simulink model "Prescan_Carsim_1110_cs"  (R2019b)
settings: Solver=ode5  StartTime=0.0  StopTime=inf  FixedStep=1/20  RelTol=1e-3
PreLoadFcn:
  | mbxruntime.callbacks.PreLoadFcn(bdroot);
PostLoadFcn:
  | mbxruntime.callbacks.PostLoadFcn(bdroot);
InitFcn:
  | mbxruntime.callbacks.InitFcn(bdroot);
  | Initialization_Func;
  | %T01_Init_2106;
StartFcn:
  | mbxruntime.callbacks.StartFcn(bdroot);
  | current_sys=gcs;
  | speedblock=Simulink.findBlocks(current_sys,'Name','speed_kmh_Gain');
  | h1=add_exec_event_listener(speedblock,'PostOutputs',@SpeedVisulization);
  | outblock=Simulink.findBlocks(current_sys,'Name','trajectorycurveoutput_Gain');
  | CurveTrajectoryListenerHandle=add_exec_event_listener(outblock,'PostOutputs',@TrajectoryCurve_CallBack);
  | lanedatablock=Simulink.findBlocks(current_sys,'Name','LaneData_Gain');
  | CurveLaneListenerHandle=add_exec_event_listener(lanedatablock,'PostOutputs',@CurveLane_CallBack);
StopFcn:
  | mbxruntime.callbacks.StopFcn(bdroot);
model workspace: external: MAT-File .\Prescan_Carsim_1110_cs_hws.mat (data not in the file)
undefined symbols (not defined in the file): AAx, AAy, AAz, AVx, AVy, AVz, Ax, Ay, Az, canChannel, DiscIntNeverNeededParam, g, InitialDPMPDF_Comfort, InitialDPMPDF_Efficiency, InitialDPMPDF_Safety, InitialPDF_DEM, InitialPlanningParameter, Kf, Kr, Lr, M, mbxruntime, nG, NormalisedTrajectoryIndicator_Pool, Parameter_Indicator_LookUpTable, Prescan_Carsim_1110_cs_119509d653dbd015, Prescan_Carsim_1110_cs_2a185a1795bc1743, Prescan_Carsim_1110_cs_518c510c1da40fb3, Prescan_Carsim_1110_cs_52de4d8fa74bbcb1, Prescan_Carsim_1110_cs_b8364abf183e6ec6, Prescan_Carsim_1110_cs_fca2a77e3ded9ac6, Rational_Coefficient_Learning, SteeringWheel, TrajectoryIndicatorRange, V, VehicleBaseLength, Vx, Vy, Vz
libraries: canmsglib x11, dsparch4 x5, canlib x3, PreScanSimulinkLibrary x3, Solver_SF x1, autolibshared x1
(part 3 of 6)

== system Prescan_Carsim_1110_cs/BMW_X5_SUV_1/LaneMarkerSensor_1_Data/If Action Subsystem2 ==
  In1 : Inport
  In2 : Inport  Port=2
  Action Port : ActionPort  ActionPortLabel=if(u1 >= u2)
  Bus Selector : BusSelector  OutputSignals=DATA
  Selector : Selector  IndexOptions=Index vector (port)  Indices=[4]  OutputSizes=1
  Out1 : Outport
  wires:
  Bus Selector/1 -> Out1/1  "<DATA>"
  Selector/1 -> Bus Selector/1
  In1/1 -> Selector/1
  In2/1 -> Selector/2

== system Prescan_Carsim_1110_cs/BMW_X5_SUV_1/LaneMarkerSensor_1_Data/If Action Subsystem3 ==
  In1 : Inport
  In2 : Inport  Port=2
  Action Port : ActionPort  ActionPortLabel=if(u1 >= u2)
  Bus Selector : BusSelector  OutputSignals=DATA
  Selector : Selector  IndexOptions=Index vector (port)  Indices=[4]  OutputSizes=1
  Out1 : Outport
  wires:
  Bus Selector/1 -> Out1/1  "<DATA>"
  Selector/1 -> Bus Selector/1
  In1/1 -> Selector/1
  In2/1 -> Selector/2

== system Prescan_Carsim_1110_cs/BMW_X5_SUV_1/LaneMarkerSensor_1_Data/If Action Subsystem4 ==
  In1 : Inport
  In2 : Inport  Port=2
  Action Port : ActionPort  ActionPortLabel=if(u1 >= u2)
  Bus Selector : BusSelector  OutputSignals=DATA
  Selector : Selector  IndexOptions=Index vector (port)  Indices=[4]  OutputSizes=1
  Out1 : Outport
  wires:
  Bus Selector/1 -> Out1/1  "<DATA>"
  Selector/1 -> Bus Selector/1
  In1/1 -> Selector/1
  In2/1 -> Selector/2

== system Prescan_Carsim_1110_cs/BMW_X5_SUV_1/SELF_Demux/compas converter ==
  rotz [rad] : Inport
  cart2compas : Subsystem
  rad2deg : Gain  Gain=180/pi
  heading [deg] : Outport
  wires:
  rad2deg/1 -> cart2compas/1(Angle [deg])
  rotz [rad]/1 -> rad2deg/1
  cart2compas/1(heading [deg]) -> heading [deg]/1

== system Prescan_Carsim_1110_cs/BMW_X5_SUV_1/Tracking Control & vehicle dynamics/Lane Keeping Assistance ==
  note: Trajectory Trackin-LQR controller, Carsim Model
  note: Trajectory Trackin-LQR controller, Simulink VDM
  note: Trajectory Tracking Controller-SMC controller
  DataUsedForTracking (PrescanToTarget)t : Inport
  Bus Selector : BusSelector  OutputSignals=Preview Error,HeadError_rad,Curvature,PreviewDistance,Speed_Kmh
  Digital Filter Design6 : dsparch4/Digital Filter Design  Commented=on  mwdsp_browser_bugfix_var=off
  From : From  Commented=on  GotoTag=SMC_c1  TagVisibility=global
  From1 : From  Commented=on  GotoTag=SMC_c2  TagVisibility=global
  From3 : From  Commented=on  GotoTag=delta  TagVisibility=global
  From4 : From  Commented=on  GotoTag=kapa  TagVisibility=global
  Gain : Gain  Gain=180/pi
  Gain1 : Gain  Gain=1/3.6
  Manual Switch : ManualSwitch  CurrentSetting=0
  Manual Switch1 : ManualSwitch  CurrentSetting=0
  Path Tracking - LQR controller : Subsystem  Commented=on
  Path Tracking - LQR controller1 : Subsystem
  Path Tracking - SMC controller : MATLAB Function  Commented=on  TreatAsAtomicUnit=on
  SMC characters : Subsystem  Commented=on
  derivative_filter : Subsystem
  "derivative_filter " : Subsystem
  steering angle_Front(deg) : Outport
  wires:
  Path Tracking - LQR controller/1(SteeringAngle_Front(rad)) -> Manual Switch1/1
  Gain1/1 -> Path Tracking - LQR controller1/7(Speed_m/s), Path Tracking - LQR controller/7(Speed_m/s), Path Tracking - SMC controller/11(v)
  Gain/1 -> steering angle_Front(deg)/1
  "derivative_filter "/1(Out1) -> Path Tracking - LQR controller1/2(PreviewError_dot), Path Tracking - LQR controller/2(PreviewError_dot), Path Tracking - SMC controller/6(PreviewError_dot)
  Digital Filter Design6/1 -> Manual Switch/1  "steering angle"
  From/1 -> Path Tracking - SMC controller/1(c1)
  derivative_filter/1(Out1) -> Path Tracking - LQR controller1/4(HeadingError_dot), Path Tracking - LQR controller/4(HeadingError_dot), Path Tracking - SMC controller/8(HeadingError_dot)
  Path Tracking - SMC controller/1(SteerAngle) -> Digital Filter Design6/1
  From3/1 -> Path Tracking - SMC controller/3(delta)
  From1/1 -> Path Tracking - SMC controller/2(c2)
  From4/1 -> Path Tracking - SMC controller/4(kapa)
  Bus Selector/5 -> Gain1/1  "<Speed_Kmh>"
  Bus Selector/1 -> Path Tracking - SMC controller/5(PreviewError), Path Tracking - LQR controller1/1(PreviewError), Path Tracking - LQR controller/1(PreviewError), "derivative_filter "/1(In1)  "<Preview Error>"
  Bus Selector/4 -> Path Tracking - SMC controller/10(PreviewDistance), Path Tracking - LQR controller1/6(Preview_Distance), Path Tracking - LQR controller/6(Preview_Distance)  "<PreviewDistance>"
  Bus Selector/2 -> Path Tracking - LQR controller1/3(HeadingError), Path Tracking - LQR controller/3(HeadingError), Path Tracking - SMC controller/7(HeadingError), derivative_filter/1(In1)  "<HeadError_rad>"
  Manual Switch/1 -> Gain/1
  Bus Selector/3 -> Path Tracking - LQR controller1/5(Curvature), Path Tracking - LQR controller/5(Curvature), Path Tracking - SMC controller/9(Curvature)  "<Curvature>"
  DataUsedForTracking (PrescanToTarget)t/1 -> Bus Selector/1
  Path Tracking - LQR controller1/1(SteeringAngle_Front(rad)) -> Manual Switch1/2
  Manual Switch1/1 -> Manual Switch/2

== system Prescan_Carsim_1110_cs/BMW_X5_SUV_1/Tracking Control & vehicle dynamics/simple_filter10 ==
  In1 : Inport
  Add : Sum
  Gain10 : Gain  Gain=0.5
  Memory : Memory
  Out1 : Outport  VectorParamsAs1DForOutWhenUnconnected=off
  wires:
  Gain10/1 -> Out1/1
  Memory/1 -> Add/2
  In1/1 -> Add/1, Memory/1
  Add/1 -> Gain10/1

== system Prescan_Carsim_1110_cs/BMW_X5_SUV_1/Tracking Control & vehicle dynamics/simple_filter11 ==
  In1 : Inport
  Add : Sum
  Gain10 : Gain  Gain=0.5
  Memory : Memory
  Out1 : Outport  VectorParamsAs1DForOutWhenUnconnected=off
  wires:
  Gain10/1 -> Out1/1
  Memory/1 -> Add/2
  In1/1 -> Add/1, Memory/1
  Add/1 -> Gain10/1

== system Prescan_Carsim_1110_cs/BMW_X5_SUV_1/Tracking Control & vehicle dynamics/simple_filter6 ==
  In1 : Inport
  Add : Sum
  Gain10 : Gain  Gain=0.5
  Memory : Memory
  Out1 : Outport  VectorParamsAs1DForOutWhenUnconnected=off
  wires:
  Add/1 -> Gain10/1
  In1/1 -> Memory/1, Add/1
  Memory/1 -> Add/2
  Gain10/1 -> Out1/1

== system Prescan_Carsim_1110_cs/BMW_X5_SUV_1/Tracking Control & vehicle dynamics/simple_filter7 ==
  In1 : Inport
  Add : Sum
  Gain10 : Gain  Gain=0.5
  Memory : Memory
  Out1 : Outport  VectorParamsAs1DForOutWhenUnconnected=off
  wires:
  Gain10/1 -> Out1/1
  Memory/1 -> Add/2
  In1/1 -> Add/1, Memory/1
  Add/1 -> Gain10/1

== system Prescan_Carsim_1110_cs/BMW_X5_SUV_1/Tracking Control & vehicle dynamics/simple_filter8 ==
  In1 : Inport
  Add : Sum
  Gain10 : Gain  Gain=0.5
  Memory : Memory
  Out1 : Outport  VectorParamsAs1DForOutWhenUnconnected=off
  wires:
  Add/1 -> Gain10/1
  In1/1 -> Memory/1, Add/1
  Memory/1 -> Add/2
  Gain10/1 -> Out1/1

== system Prescan_Carsim_1110_cs/BMW_X5_SUV_1/Tracking Control & vehicle dynamics/simple_filter9 ==
  In1 : Inport
  Add : Sum
  Gain10 : Gain  Gain=0.5
  Memory : Memory
  Out1 : Outport  VectorParamsAs1DForOutWhenUnconnected=off
  wires:
  Gain10/1 -> Out1/1
  Memory/1 -> Add/2
  In1/1 -> Add/1, Memory/1
  Add/1 -> Gain10/1

== system Prescan_Carsim_1110_cs/BMW_X5_SUV_1/Trajectory Indicator Calculation/VehicleInfo_Curve ==
  In1 : Inport
  Trigger : TriggerPort  TriggerType=falling  VariantControl=Variant
  trajectorycurveoutput_Gain : Gain
  VehicleInfo_Curve : Outport
  wires:
  In1/1 -> trajectorycurveoutput_Gain/1
  trajectorycurveoutput_Gain/1 -> VehicleInfo_Curve/1

== system Prescan_Carsim_1110_cs/BMW_X5_SUV_1/Trajectory Indicator Calculation/VehicleState_Buffer ==
  In1 : Inport
  Enable : EnablePort  StatesWhenEnabling=reset  PropagateVarSize=During execution
  VehicleInfo_StoreDuringCurve : MATLAB Function  TreatAsAtomicUnit=on
  VehicleInfo_Curve : Outport
  wires:
  In1/1 -> VehicleInfo_StoreDuringCurve/1(VehicleState_Var)
  VehicleInfo_StoreDuringCurve/1(VehicleState_Curve) -> VehicleInfo_Curve/1

== system Prescan_Carsim_1110_cs/BMW_X5_SUV_1/VehicleToPrescan/simple_filter10 ==
  In1 : Inport
  Add : Sum
  Gain10 : Gain  Gain=0.5
  Memory : Memory
  Out1 : Outport  VectorParamsAs1DForOutWhenUnconnected=off
  wires:
  Gain10/1 -> Out1/1
  Memory/1 -> Add/2
  In1/1 -> Add/1, Memory/1
  Add/1 -> Gain10/1

== system Prescan_Carsim_1110_cs/BMW_X5_SUV_1/VehicleToPrescan/simple_filter11 ==
  In1 : Inport
  Add : Sum
  Gain10 : Gain  Gain=0.5
  Memory : Memory
  Out1 : Outport  VectorParamsAs1DForOutWhenUnconnected=off
  wires:
  Gain10/1 -> Out1/1
  Memory/1 -> Add/2
  In1/1 -> Add/1, Memory/1
  Add/1 -> Gain10/1

== system Prescan_Carsim_1110_cs/BMW_X5_SUV_1/VehicleToPrescan/simple_filter6 ==
  In1 : Inport
  Add : Sum
  Gain10 : Gain  Gain=0.5
  Memory : Memory
  Out1 : Outport  VectorParamsAs1DForOutWhenUnconnected=off
  wires:
  Add/1 -> Gain10/1
  In1/1 -> Memory/1, Add/1
  Memory/1 -> Add/2
  Gain10/1 -> Out1/1

== system Prescan_Carsim_1110_cs/BMW_X5_SUV_1/VehicleToPrescan/simple_filter7 ==
  In1 : Inport
  Add : Sum
  Gain10 : Gain  Gain=0.5
  Memory : Memory
  Out1 : Outport  VectorParamsAs1DForOutWhenUnconnected=off
  wires:
  Gain10/1 -> Out1/1
  Memory/1 -> Add/2
  In1/1 -> Add/1, Memory/1
  Add/1 -> Gain10/1

== system Prescan_Carsim_1110_cs/BMW_X5_SUV_1/VehicleToPrescan/simple_filter8 ==
  In1 : Inport
  Add : Sum
  Gain10 : Gain  Gain=0.5
  Memory : Memory
  Out1 : Outport  VectorParamsAs1DForOutWhenUnconnected=off
  wires:
  Add/1 -> Gain10/1
  In1/1 -> Memory/1, Add/1
  Memory/1 -> Add/2
  Gain10/1 -> Out1/1

== system Prescan_Carsim_1110_cs/BMW_X5_SUV_1/VehicleToPrescan/simple_filter9 ==
  In1 : Inport
  Add : Sum
  Gain10 : Gain  Gain=0.5
  Memory : Memory
  Out1 : Outport  VectorParamsAs1DForOutWhenUnconnected=off
  wires:
  Gain10/1 -> Out1/1
  Memory/1 -> Add/2
  In1/1 -> Add/1, Memory/1
  Add/1 -> Gain10/1

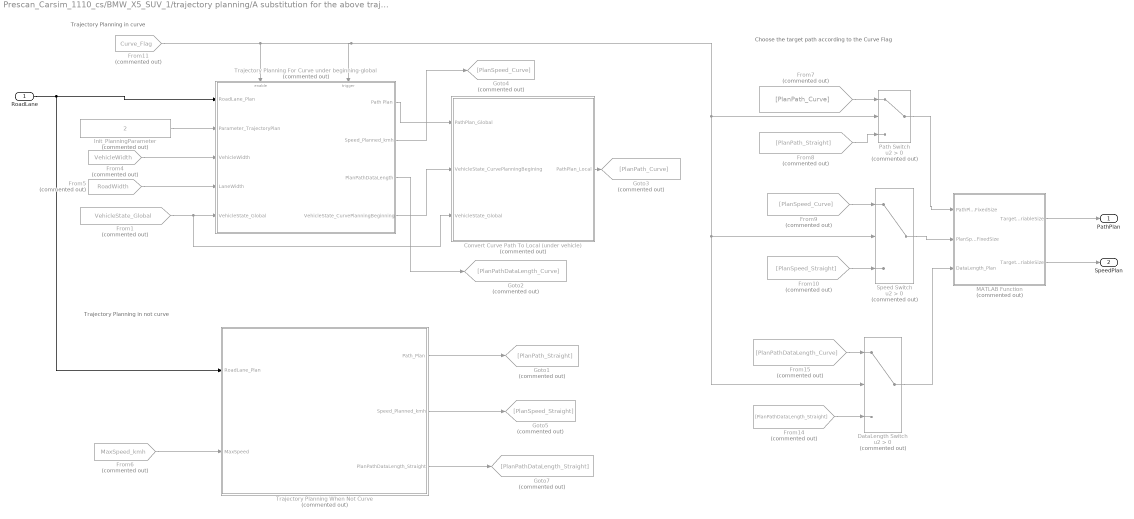
== system Prescan_Carsim_1110_cs/BMW_X5_SUV_1/trajectory planning/A substitution for the above trajectory planning subsystem ==
  note: Choose the target path according to the Curve Flag
  note: Trajectory Planning in not curve
  note: Trajectory Planning in curve
  RoadLane : Inport
  Convert Curve Path To Local (under vehicle) : MATLAB Function  Commented=on  TreatAsAtomicUnit=on
  DataLength Switch : Switch  Commented=on  Criteria=u2 > Threshold
  From1 : From  Commented=on  GotoTag=VehicleState_Global  TagVisibility=global
  From10 : From  Commented=on  GotoTag=PlanSpeed_Straight
  From11 : From  Commented=on  GotoTag=Curve_Flag  TagVisibility=global
  From14 : From  Commented=on  GotoTag=PlanPathDataLength_Straight
  From15 : From  Commented=on  GotoTag=PlanPathDataLength_Curve
  From4 : From  Commented=on  GotoTag=VehicleWidth  TagVisibility=global
  From5 : From  Commented=on  GotoTag=RoadWidth  TagVisibility=global
  From6 : From  Commented=on  GotoTag=MaxSpeed_kmh  TagVisibility=global
  From7 : From  Commented=on  GotoTag=PlanPath_Curve
  From8 : From  Commented=on  GotoTag=PlanPath_Straight
  From9 : From  Commented=on  GotoTag=PlanSpeed_Curve
  Goto1 : Goto  Commented=on  GotoTag=PlanPath_Straight
      settings: AttributesFormatString=output:fixed size,1000*2
  Goto2 : Goto  Commented=on  GotoTag=PlanPathDataLength_Curve
  Goto3 : Goto  Commented=on  GotoTag=PlanPath_Curve
      settings: AttributesFormatString=|
      | Path local under the vehicle
      | output:fixed size 1000*2
  Goto4 : Goto  Commented=on  GotoTag=PlanSpeed_Curve
      settings: AttributesFormatString=The size is fixed 1000*1
  Goto5 : Goto  Commented=on  GotoTag=PlanSpeed_Straight
      settings: AttributesFormatString=The size vas fixed 1000*1
  Goto7 : Goto  Commented=on  GotoTag=PlanPathDataLength_Straight
      settings: AttributesFormatString=|
      | Used to extract the valid
      | PlanPath data
  Init_PlanningParameter : Constant  Commented=on  Value=2
  MATLAB Function : MATLAB Function  Commented=on  TreatAsAtomicUnit=on  SystemSampleTime=1/20
      settings: AttributesFormatString=|
      | Convert Variable Size into Fixed Size
      | Specified Sample Time:1/20
  Path Switch : Switch  Commented=on  Criteria=u2 > Threshold
  Speed Switch : Switch  Commented=on  Criteria=u2 > Threshold
  Trajectory Planning For Curve under beginning-global : Subsystem  Commented=on
  Trajectory Planning When Not Curve : MATLAB Function  Commented=on  TreatAsAtomicUnit=on
  PathPlan : Outport
  SpeedPlan : Outport  Port=2
  wires:
  From9/1 -> Speed Switch/1
  From11/1 -> Trajectory Planning For Curve under beginning-global/Trigger, Speed Switch/2, DataLength Switch/2, Path Switch/2, Trajectory Planning For Curve under beginning-global/Enable
  Trajectory Planning For Curve under beginning-global/2(Speed_Planned_kmh) -> Goto4/1
  From15/1 -> DataLength Switch/1
  Path Switch/1 -> MATLAB Function/1(PathPlan_FixedSize)
  DataLength Switch/1 -> MATLAB Function/3(DataLength_Plan)
  From10/1 -> Speed Switch/3
  From14/1 -> DataLength Switch/3
  From8/1 -> Path Switch/3
  Speed Switch/1 -> MATLAB Function/2(PlanSpeed_FixedSize)
  Trajectory Planning When Not Curve/3(PlanPathDataLength_Straight) -> Goto7/1
  Trajectory Planning For Curve under beginning-global/3(PlanPathDataLength) -> Goto2/1
  Trajectory Planning For Curve under beginning-global/1(Path Plan) -> Convert Curve Path To Local (under vehicle)/1(PathPlan_Global)
  From1/1 -> Trajectory Planning For Curve under beginning-global/5(VehicleState_Global), Convert Curve Path To Local (under vehicle)/3(VehicleState_Global)
  Trajectory Planning For Curve under beginning-global/4(VehicleState_CurvePlanningBeginning) -> Convert Curve Path To Local (under vehicle)/2(VehicleState_CurvePlanningBegining)
  Init_PlanningParameter/1 -> Trajectory Planning For Curve under beginning-global/2(Parameter_TrajectoryPlan)
  RoadLane/1 -> Trajectory Planning When Not Curve/1(RoadLane_Plan), Trajectory Planning For Curve under beginning-global/1(RoadLane_Plan)
  Trajectory Planning When Not Curve/2(Speed_Planned_kmh) -> Goto5/1
  From7/1 -> Path Switch/1
  From5/1 -> Trajectory Planning For Curve under beginning-global/4(LaneWidth)
  From4/1 -> Trajectory Planning For Curve under beginning-global/3(VehicleWidth)
  Trajectory Planning When Not Curve/1(Path_Plan) -> Goto1/1
  Convert Curve Path To Local (under vehicle)/1(PathPlan_Local) -> Goto3/1
  From6/1 -> Trajectory Planning When Not Curve/2(MaxSpeed)
  MATLAB Function/1(TargetPath_VariableSize) -> PathPlan/1
  MATLAB Function/2(TargetSpeed_VariableSize) -> SpeedPlan/1

== system Prescan_Carsim_1110_cs/BMW_X5_SUV_1/trajectory planning/Generate Road Lane from Polyfit TLC calculation  ==
  PolyRoadLane : Inport
  RoadLaneEnd_Rotation : Inport  Port=2
  Mux : Mux  Inputs=2
  Pre_Dis : Constant  Value=150
      settings: AttributesFormatString=The Preview Distance used to calculate the TLC
  Scope : Scope
  "TLC calculation and Lane Generation Road Lane " : MATLAB Function  TreatAsAtomicUnit=on
      settings: AttributesFormatString=|
      | The TLC could not be calculated because
      | of the optimal function is not available
      | for simulink code generation
  Terminator : Terminator
  tag scope: TLC_Left=global, TLC_Right=global
  wires:
  PolyRoadLane/1 -> "TLC calculation and Lane Generation Road Lane "/1(PolyRoadLane)
  "TLC calculation and Lane Generation Road Lane "/2(TLC_Left) -> Mux/1, [TLC_Left]
  [Interval_RoadSegment] -> "TLC calculation and Lane Generation Road Lane "/3(IntervalRoadSegment)
  RoadLaneEnd_Rotation/1 -> "TLC calculation and Lane Generation Road Lane "/2(RoadLaneEnd_Rotation)
  [RoadWidth] -> "TLC calculation and Lane Generation Road Lane "/4(Width_Road)
  [VehicleWidth] -> "TLC calculation and Lane Generation Road Lane "/5(Width_Vehicle)
  Pre_Dis/1 -> "TLC calculation and Lane Generation Road Lane "/7(Range)
  [VehicleBaseLength] -> "TLC calculation and Lane Generation Road Lane "/6(Length_Vehicle)
  [YawRate] -> "TLC calculation and Lane Generation Road Lane "/8(YawRate)
  [Speed_Rel] -> "TLC calculation and Lane Generation Road Lane "/9(Speed)
  "TLC calculation and Lane Generation Road Lane "/3(TLC_Right) -> Mux/2, [TLC_Right]
  "TLC calculation and Lane Generation Road Lane "/1(RoadLane_Plan) -> Terminator/1
  Mux/1 -> Scope/1

== system Prescan_Carsim_1110_cs/BMW_X5_SUV_1/trajectory planning/Out of Specific Curve Planning ==
  RoadLane_Plan : Inport
  MaxSpeed_Kmh : Inport  Port=2
  Action Port : ActionPort  ActionPortLabel=else
  Trajectory Planning When Not Curve : MATLAB Function  TreatAsAtomicUnit=on
  Path Plan : Outport
  Speed_Planned_kmh : Outport  Port=2
  PlanPathDataLength : Outport  Port=3
  wires:
  RoadLane_Plan/1 -> Trajectory Planning When Not Curve/1(RoadLane_Plan)
  Trajectory Planning When Not Curve/1(Path_Plan) -> Path Plan/1
  Trajectory Planning When Not Curve/2(Speed_Planned_kmh) -> Speed_Planned_kmh/1
  Trajectory Planning When Not Curve/3(PlanPathDataLength_Straight) -> PlanPathDataLength/1
  MaxSpeed_Kmh/1 -> Trajectory Planning When Not Curve/2(MaxSpeed)

== system Prescan_Carsim_1110_cs/BMW_X5_SUV_1/trajectory planning/Specific Curve Trajectory Planning ==
  CurveFlag : Inport
  RoadLane_Plan : Inport  Port=2
  PlanningParameter : Inport  Port=3
  VehicleWidth : Inport  Port=4
  LaneWidth : Inport  Port=5
  VehicleState_Global : Inport  Port=6
  Action Port : ActionPort  InitializeStates=reset  PropagateVarSize=During execution  ActionPortLabel=if(u1 > 0)
  Convert Curve Path To Local (under vehicle) : MATLAB Function  TreatAsAtomicUnit=on
  Trajectory Planning For Curve under beginning-global : Subsystem
  Path Plan : Outport
  Speed_Planned_kmh : Outport  Port=2
  PlanPathDataLength : Outport  Port=3
  wires:
  CurveFlag/1 -> Trajectory Planning For Curve under beginning-global/Trigger
  Trajectory Planning For Curve under beginning-global/1(Path Plan) -> Convert Curve Path To Local (under vehicle)/1(PathPlan_Global)
  Convert Curve Path To Local (under vehicle)/1(PathPlan_Local) -> Path Plan/1
  Trajectory Planning For Curve under beginning-global/2(Speed_Planned_kmh) -> Speed_Planned_kmh/1
  Trajectory Planning For Curve under beginning-global/3(PlanPathDataLength) -> PlanPathDataLength/1
  RoadLane_Plan/1 -> Trajectory Planning For Curve under beginning-global/1(RoadLane_Plan)
  VehicleState_Global/1 -> Trajectory Planning For Curve under beginning-global/5(VehicleState_Global), Convert Curve Path To Local (under vehicle)/2(VehicleState_Global)
  VehicleWidth/1 -> Trajectory Planning For Curve under beginning-global/3(VehicleWidth)
  LaneWidth/1 -> Trajectory Planning For Curve under beginning-global/4(LaneWidth)
  PlanningParameter/1 -> Trajectory Planning For Curve under beginning-global/2(Parameter_TrajectoryPlan)

== system Prescan_Carsim_1110_cs/BMW_X5_SUV_1/trajectory planning/Subsystem ==
  Choose curve length for different curve No : MultiPortSwitch  Inputs=4  DataPortForDefault=Additional data port  DiagnosticForDefault=None
  Constant : Constant
  Constant1 : Constant  Value=0
  "Curve 1 " : Constant  Value=308
  Curve 2 : Constant  Value=308
  Curve 3 : Constant  Value=308
  Curve 4 : Constant  Value=308
  Determination of Curve Road No : Subsystem
  Not Curve : Constant  Value=160
  Sum : Sum  Inputs=2
  Switch : Switch  Criteria=u2 > Threshold  Threshold=0.5
  The planned path length after curve : Constant  Value=8
      settings: AttributesFormatString=Should consider the Preview Distance
  Expected PathPlanning Length : Outport
  Curve Flag : Outport  Port=2
      settings: AttributesFormatString=|
      | 1: Curve
      | 0: Not Curve
  wires:
  Determination of Curve Road No/1(Curve No) -> Switch/2, Choose curve length for different curve No/1
  Not Curve/1 -> Choose curve length for different curve No/6
  Curve 4/1 -> Choose curve length for different curve No/5
  Curve 3/1 -> Choose curve length for different curve No/4
  Sum/1 -> Expected PathPlanning Length/1
  Curve 2/1 -> Choose curve length for different curve No/3
  "Curve 1 "/1 -> Choose curve length for different curve No/2
  The planned path length after curve/1 -> Sum/2
  Choose curve length for different curve No/1 -> Sum/1
  Switch/1 -> Curve Flag/1
  Constant/1 -> Switch/1
  Constant1/1 -> Switch/3

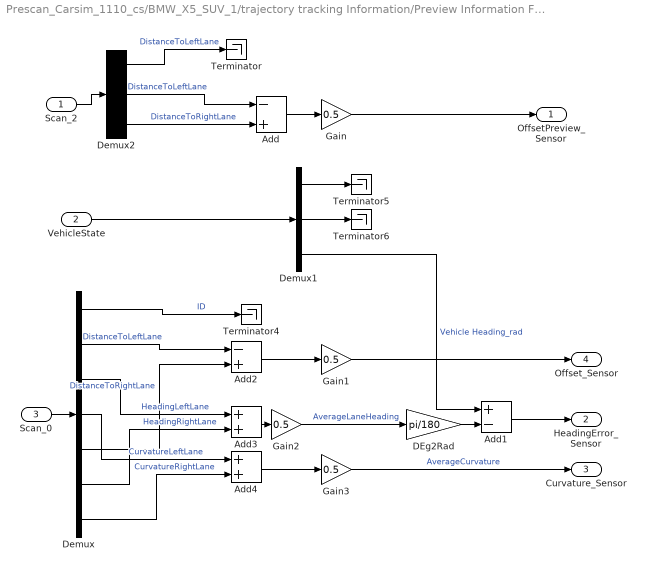
== system Prescan_Carsim_1110_cs/BMW_X5_SUV_1/trajectory tracking Information/Preview Information From LaneMarkerSensor ==
  Scan_2 : Inport
  VehicleState : Inport  Port=2
  Scan_0 : Inport  Port=3
  Add : Sum  Inputs=-+
  Add1 : Sum  Inputs=+-
  Add2 : Sum  Inputs=-+
  Add3 : Sum
  Add4 : Sum
  DEg2Rad : Gain  Gain=pi/180
  Demux : Demux  Outputs=7  BusSelectionMode=on
  Demux1 : Demux  Outputs=3
  Demux2 : Demux  Outputs=3  BusSelectionMode=on
  Gain{,1..3} (4 alike) : Gain  Gain=0.5
  Terminator{,4..6} (4 alike) : Terminator
  OffsetPreview_Sensor : Outport
  HeadingError_Sensor : Outport  Port=2
  Curvature_Sensor : Outport  Port=3
  Offset_Sensor : Outport  Port=4
  wires:
  Add1/1 -> HeadingError_Sensor/1
  Demux1/1 -> Terminator5/1
  VehicleState/1 -> Demux1/1
  Scan_0/1 -> Demux/1
  Demux1/2 -> Terminator6/1
  Scan_2/1 -> Demux2/1
  Demux2/3 -> Add/2  "DistanceToRightLane"
  Demux2/2 -> Add/1  "DistanceToLeftLane"
  Gain/1 -> OffsetPreview_Sensor/1
  Demux1/3 -> Add1/1  "Vehicle Heading_rad"
  Demux/2 -> Add2/1  "DistanceToLeftLane"
  Gain1/1 -> Offset_Sensor/1
  Add2/1 -> Gain1/1
  Demux/1 -> Terminator4/1  "ID"
  Add3/1 -> Gain2/1
  Gain2/1 -> DEg2Rad/1  "AverageLaneHeading"
  Demux/6 -> Add3/2  "HeadingRightLane"
  Demux/7 -> Add4/2  "CurvatureRightLane"
  Demux/5 -> Add2/2  "DistanceToRightLane"
  Demux/4 -> Add4/1  "CurvatureLeftLane"
  Add4/1 -> Gain3/1
  Demux/3 -> Add3/1  "HeadingLeftLane"
  Gain3/1 -> Curvature_Sensor/1  "AverageCurvature"
  Add/1 -> Gain/1
  Demux2/1 -> Terminator/1  "DistanceToLeftLane"
  DEg2Rad/1 -> Add1/2

== system Prescan_Carsim_1110_cs/SteeringWheel_pivot_BMW_X5_SUV_1/Actuator/visu_Rotate ==
  In1 : Inport
  sfun_RPYActuator : S-Function  FunctionName=sfun_RPYActuator  Parameters=SParameter1, SParameter2, SampleTime  SFunctionDeploymentMode=off  EnableBusSupport=off  mask(Legacy Function){SFunctionSpec=void prescan_outputFcn(void ** work1,  PRESCAN_XYZ_DATA u1[1]), SParameter1=UniqueID, SParameter2=uint8([Object3DID 0]), SampleTime=TimeStep, ShowSpec=on}
      mask prompts: SParameter1 "P1:"; SParameter2 "P2:"; SampleTime "Sample time (-1 for inherited):"; ShowSpec "Display function specification"
      mask help:
      | This block allows you to call the legacy functions specified by the following Legacy Code Tool definition:
      | def.SFunctionName = 'sfun_PositionActuator';
      | def.OutputFcnSpec = 'void prescan_outputFcn(void ** work1,  PRESCAN_XYZ_DATA u1[1])';
      | def.StartFcnSpec = 'void prescan_startFcn(void ** work1, uint8 p1[], double p2)';
      | def.TerminateFcnSpec = 'void prescan_terminateFcn(void ** work1)';
      | def.HeaderFiles = {'prescan_positionactuator_data.h', 'prescan_header_data.h', 'prescan_SFunLibrary.h', 'prescan_CreateLogHandler.h', 'prescan_CreateErrorHandler.h'};
      | def.SourceFiles = {'prescan_MexLogHandler.cpp', 'prescan_SimStructErrorHandler.cpp', 'prescan_ConcurrentLogHandler.cpp', 'prescan_ConcurrentErrorHandler.cpp'};
      | def.HostLibFiles = {'sensorinterfaced.lib'};
      | def.TargetLibFiles = {'sensorinterfaced.so'};
      | def.IncPaths = {'.', 'C:\prescandev\vislibrary\vis\..\pimp\include\sensors\InterfaceRTW'};
      | def.SrcPaths = {'.'};
      | def.LibPaths = {'C:\\prescandev\\vislibrary_build\lib'};
      | def.SampleTime = 'parameterized';
      mask Help: <p>This block was generated automatically by the Legacy Code Tool. For detailed help on this tool, call<a href="matlab:legacy_code('help')"> legacy_code('help')</a>.</p>
      mask Callback ShowSpec:
      | if strcmp(get_param(gcbh, 'ShowSpec'), 'on')
      |   set_param(gcbh, 'MaskDisplay', sprintf('fprintf(''%s'');', get_param(gcbh, 'SFunctionSpec')));
      | else
      |   set_param(gcbh, 'MaskDisplay', sprintf('fprintf(''%s'');', get_param(gcbh, 'FunctionName')));
      | end
      mask Display: fprintf('void prescan_outputFcn(void ** work1,  PRESCAN_XYZ_DATA u1[1])');
  wires:
  In1/1 -> sfun_RPYActuator/1

== system Prescan_Carsim_1110_cs/SteeringWheel_pivot_BMW_X5_SUV_1/Actuator/visu_Translate ==
  In1 : Inport
  sfun_PositionActuator : S-Function  FunctionName=sfun_PositionActuator  Parameters=SParameter1, SParameter2, SampleTime  SFunctionDeploymentMode=off  EnableBusSupport=off  mask(Legacy Function){SFunctionSpec=void prescan_outputFcn(void ** work1,  PRESCAN_XYZ_DATA u1[1]), SParameter1=uint8([Object3DID 0]), SParameter2=UniqueID, SampleTime=TimeStep, ShowSpec=on}
      mask prompts: SParameter1 "P1:"; SParameter2 "P2:"; SampleTime "Sample time (-1 for inherited):"; ShowSpec "Display function specification"
      mask help:
      | This block allows you to call the legacy functions specified by the following Legacy Code Tool definition:
      | def.SFunctionName = 'sfun_PositionActuator';
      | def.OutputFcnSpec = 'void prescan_outputFcn(void ** work1,  PRESCAN_XYZ_DATA u1[1])';
      | def.StartFcnSpec = 'void prescan_startFcn(void ** work1, uint8 p1[], double p2)';
      | def.TerminateFcnSpec = 'void prescan_terminateFcn(void ** work1)';
      | def.HeaderFiles = {'prescan_positionactuator_data.h', 'prescan_header_data.h', 'prescan_SFunLibrary.h', 'prescan_CreateLogHandler.h', 'prescan_CreateErrorHandler.h'};
      | def.SourceFiles = {'prescan_MexLogHandler.cpp', 'prescan_SimStructErrorHandler.cpp', 'prescan_ConcurrentLogHandler.cpp', 'prescan_ConcurrentErrorHandler.cpp'};
      | def.HostLibFiles = {'sensorinterfaced.lib'};
      | def.TargetLibFiles = {'sensorinterfaced.so'};
      | def.IncPaths = {'.', 'C:\prescandev\vislibrary\vis\..\pimp\include\sensors\InterfaceRTW'};
      | def.SrcPaths = {'.'};
      | def.LibPaths = {'C:\\prescandev\\vislibrary_build\lib'};
      | def.SampleTime = 'parameterized';
      mask Help: <p>This block was generated automatically by the Legacy Code Tool. For detailed help on this tool, call<a href="matlab:legacy_code('help')"> legacy_code('help')</a>.</p>
      mask Callback ShowSpec:
      | if strcmp(get_param(gcbh, 'ShowSpec'), 'on')
      |   set_param(gcbh, 'MaskDisplay', sprintf('fprintf(''%s'');', get_param(gcbh, 'SFunctionSpec')));
      | else
      |   set_param(gcbh, 'MaskDisplay', sprintf('fprintf(''%s'');', get_param(gcbh, 'FunctionName')));
      | end
      mask Display: fprintf('void prescan_outputFcn(void ** work1,  PRESCAN_XYZ_DATA u1[1])');
  wires:
  In1/1 -> sfun_PositionActuator/1

== system Prescan_Carsim_1110_cs/BMW_X5_SUV_1/DEM updating and Preference Estimation/UpdateDEM/Construct Comparison Group ==
  FeedBack_FromDriver : Inport
  TrajectoryIndicator : Inport  Port=2
  Comparison Group_1 : MATLAB Function  TreatAsAtomicUnit=on
  Constant : Constant  Value=NormalisedTrajectoryIndicator_Pool
  Constant7 : Constant  Value=TrajectoryIndicatorRange
  FeedBack : Outport
  Query_Normalized : Outport  Port=2
  Evaluated_NormlisedTrajectoryIndicator : Outport  Port=3
  LastPreference_Normalised : Outport  Port=4
  wires:
  Comparison Group_1/2(Query_Compare) -> Query_Normalized/1
  FeedBack_FromDriver/1 -> Comparison Group_1/1(Feedback_Driver)
  TrajectoryIndicator/1 -> Comparison Group_1/2(Real_Trajectory_Indicator)
  Constant7/1 -> Comparison Group_1/3(TrajectoryIndicatorRange)
  Constant/1 -> Comparison Group_1/4(NormalisedTrajectoryIndicator_Pool)
  Comparison Group_1/1(FeedBack) -> FeedBack/1
  Comparison Group_1/3(Evaluated_NormalisedTrajectoryIndicator) -> Evaluated_NormlisedTrajectoryIndicator/1
  Comparison Group_1/4(LastPreference_Normalised) -> LastPreference_Normalised/1

== system Prescan_Carsim_1110_cs/BMW_X5_SUV_1/DEM updating and Preference Estimation/UpdateDEM/Online DEM updating ==
  FeedBack : Inport
  Query_Compare : Inport  Port=2
  PriorPDF_DEM : Inport  Port=3
  PriorDPMPDF_Safety : Inport  Port=4
  PriorDPMPDF_Comfort : Inport  Port=5
  PriorDPMPDF_Efficiency : Inport  Port=6
  Evaluated_Normalised : Inport  Port=7
  LastPreference_NormalisedTrajectoryIndicator : Inport  Port=8
  Constant : Constant  Value=NormalisedTrajectoryIndicator_Pool
  Constant3 : Constant  Value=Rational_Coefficient_Learning
  "Select the Next Trajectory " : MATLAB Function  TreatAsAtomicUnit=on
  UPdate DEM : MATLAB Function  TreatAsAtomicUnit=on
  Next_ExpectedTrajectoryIndicator : Outport
  Next_ExpectedTrajectoryID : Outport  Port=2
  wires:
  FeedBack/1 -> UPdate DEM/1(FeedBack)
  Query_Compare/1 -> UPdate DEM/2(Query)
  PriorPDF_DEM/1 -> UPdate DEM/3(PriorPDF_DEM)
  PriorDPMPDF_Safety/1 -> UPdate DEM/4(PriorDPMPDF_Safety)
  PriorDPMPDF_Comfort/1 -> UPdate DEM/5(PriorDPMPDF_Comfort)
  PriorDPMPDF_Efficiency/1 -> UPdate DEM/6(PriorDPMPDF_Efficiency)
  Constant3/1 -> "Select the Next Trajectory "/8(Rational_Coefficient_Learning), UPdate DEM/7(Rational_Coefficient_Learning)
  UPdate DEM/1(PostPDF_DEM) -> "Select the Next Trajectory "/1(PriorPDF_DEM)
  UPdate DEM/2(PostDPMPDF_Safety) -> "Select the Next Trajectory "/2(PriorDPMPDF_Safety)
  UPdate DEM/3(PostDPMPDF_Comfort) -> "Select the Next Trajectory "/3(PriorDPMPDF_Comfort)
  UPdate DEM/4(PostDPMPDF_Effociency) -> "Select the Next Trajectory "/4(PriorDPMPDF_Efficiency)
  "Select the Next Trajectory "/2(ExpectedNext_QueryID) -> Next_ExpectedTrajectoryID/1
  "Select the Next Trajectory "/1(ExpectedNext_NormalisedTrajectoryIndicator) -> Next_ExpectedTrajectoryIndicator/1
  Constant/1 -> "Select the Next Trajectory "/5(NormalisedTrajectoryIndicator_Pool)
  Evaluated_Normalised/1 -> "Select the Next Trajectory "/6(Evaluated_NormalisedTrajectoryIndicator)
  LastPreference_NormalisedTrajectoryIndicator/1 -> "Select the Next Trajectory "/7(LastPreference_NormalisedTrajectoryIndicator)

== system Prescan_Carsim_1110_cs/BMW_X5_SUV_1/DEM updating and Preference Estimation/UpdateDEM/Trajectory Planning Parameter Management1 ==
  Expected_TrajectoryIndicators : Inport
  ExpectedNext_QueryID : Inport  Port=2
  Constant : Constant  Value=InitialPlanningParameter
  Constant4 : Constant  Value=Parameter_Indicator_LookUpTable
  Determine planning parameter according to the expected TrajectoryIndicators_LookUpTable : MATLAB Function  TreatAsAtomicUnit=on
  From : From  Commented=on  GotoTag=Parameter_Indicator_LookUpTable  TagVisibility=global
  From2 : From  Commented=on  GotoTag=InitialPlanningParameter  TagVisibility=global
  Trajectory parameter : Outport
  wires:
  Expected_TrajectoryIndicators/1 -> Determine planning parameter according to the expected TrajectoryIndicators_LookUpTable/2(unused)
  ExpectedNext_QueryID/1 -> Determine planning parameter according to the expected TrajectoryIndicators_LookUpTable/3(ExpectedNext_QueryID)
  Determine planning parameter according to the expected TrajectoryIndicators_LookUpTable/1(PlanningParameter) -> Trajectory parameter/1
  Constant/1 -> Determine planning parameter according to the expected TrajectoryIndicators_LookUpTable/1(IntialTrajectoryPlanningParameter)
  Constant4/1 -> Determine planning parameter according to the expected TrajectoryIndicators_LookUpTable/4(Parameter_IndicatorLookUpTable)

== system Prescan_Carsim_1110_cs/BMW_X5_SUV_1/DEM updating and Preference Estimation/UpdateDEM/Trajectory Planning Parameter Management2 ==
  Expected_TrajectoryIndicators : Inport
  Next_ExpectedTrajectoryIndicatorID : Inport  Port=2
  Constant4 : Constant  Value=Parameter_Indicator_LookUpTable
  Determine planning parameter according to the expected TrajectoryIndicators_LookUpTable : MATLAB Function  TreatAsAtomicUnit=on
  Trajectory parameter : Outport
  wires:
  Expected_TrajectoryIndicators/1 -> Determine planning parameter according to the expected TrajectoryIndicators_LookUpTable/1(unused)
  Next_ExpectedTrajectoryIndicatorID/1 -> Determine planning parameter according to the expected TrajectoryIndicators_LookUpTable/2(ExpectedNext_QueryID)
  Determine planning parameter according to the expected TrajectoryIndicators_LookUpTable/1(PlanningParameter) -> Trajectory parameter/1
  Constant4/1 -> Determine planning parameter according to the expected TrajectoryIndicators_LookUpTable/3(Parameter_IndicatorLookUpTable)

== system Prescan_Carsim_1110_cs/BMW_X5_SUV_1/DEM updating and Preference Estimation/UpdateDEM/online DPM building preference estimation accordign to feedback ==
  note: DEM-
      | Update the DEM and Estimate the Preference
  feedback : Inport
  Trajectory_Indicators : Inport  Port=2
  " Driver Perception Model preference to trajectory indicator" : Subsystem  Commented=on
  Constant : Constant  Value=NormalisedTrajectoryIndicator_Pool
  Constant1 : Constant  Value=InitialPDF_DEM
      settings: AttributesFormatString=|
      | The Initial probability density Distribution
      | of the S-C-E weight of the DEM
  Constant2 : Constant  Value=InitialDPMPDF_Safety
      settings: AttributesFormatString=|
      | The Initial probability density Distribution
      | of the DPM for S-C-E
  Constant3 : Constant  Value=Rational_Coefficient_Learning
  Constant5 : Constant  Value=InitialDPMPDF_Comfort
      settings: AttributesFormatString=|
      | The Initial probability density Distribution
      | of the DPM for S-C-E
  Constant6 : Constant  Value=InitialDPMPDF_Efficiency
      settings: AttributesFormatString=|
      | The Initial probability density Distribution
      | of the DPM for S-C-E
  Constant7 : Constant  Value=TrajectoryIndicatorRange
  MATLAB Function : MATLAB Function  TreatAsAtomicUnit=on
  Terminator{,1..3} (4 alike) : Terminator
  Expected_TrajectoryIndicators : Outport
  ExpectedNext_QueryID : Outport  Port=2
  wires:
  MATLAB Function/1(ExpectedNext_NormalisedTrajectoryIndicator) -> Expected_TrajectoryIndicators/1
  MATLAB Function/2(ExpectedNext_QueryID) -> ExpectedNext_QueryID/1
  MATLAB Function/6(PostDPMPDF_Effociency) -> Terminator3/1
  MATLAB Function/5(PostDPMPDF_Comfort) -> Terminator2/1
  Constant7/1 -> MATLAB Function/8(TrajectoryIndicatorRange)
  Constant6/1 -> MATLAB Function/7(InitialDPMPDF_Efficiency)
  Constant5/1 -> MATLAB Function/6(InitialDPMPDF_Comfort)
  MATLAB Function/4(PostDPMPDF_Safety) -> Terminator1/1
  MATLAB Function/3(PostPDF_DEM) -> Terminator/1
  Trajectory_Indicators/1 -> MATLAB Function/2(Real_Trajectory_Indicator)
  Constant3/1 -> MATLAB Function/9(Rational_Coefficient_Learning)
  Constant2/1 -> MATLAB Function/5(InitialDPMPDF_Safety)
  Constant1/1 -> MATLAB Function/4(InitialPDF_DEM)
  Constant/1 -> MATLAB Function/3(NormalisedTrajectoryIndicator_Pool)
  feedback/1 -> MATLAB Function/1(FeedBack)

== system Prescan_Carsim_1110_cs/BMW_X5_SUV_1/DriverFeedBack/Generate the FeedBack Obtainment Trigger Signal/Subsystem ==
  In1 : Inport
  Trigger : TriggerPort  TriggerType=falling  VariantControl=Variant  PortDimensions=1
  Beginning Time : Outport
  wires:
  In1/1 -> Beginning Time/1

== system Prescan_Carsim_1110_cs/BMW_X5_SUV_1/SELF_Demux/compas converter/cart2compas ==
  Angle [deg] : Inport
  Constant : Constant  Value=90
  Constant1 : Constant  Value=360
  Gain : Gain  Gain=1/360
  Gain1 : Gain  Gain=360
  Gain2 : Gain  Gain=-1
  Rounding Function : Rounding
  Sum : Sum  Inputs=|-+
  Sum1 : Sum  Inputs=-+|
  Sum2 : Sum  Inputs=++|
  heading [deg] : Outport
  wires:
  Gain/1 -> Rounding Function/1
  Rounding Function/1 -> Gain1/1
  Gain1/1 -> Sum/1
  Angle [deg]/1 -> Sum1/2
  Sum/1 -> Gain2/1
  Sum1/1 -> Gain/1, Sum/2
  Constant/1 -> Sum1/1
  Gain2/1 -> Sum2/2
  Constant1/1 -> Sum2/1
  Sum2/1 -> heading [deg]/1

== system Prescan_Carsim_1110_cs/BMW_X5_SUV_1/Tracking Control & vehicle dynamics/Lane Keeping Assistance/Path Tracking - LQR controller ==
  PreviewError : Inport
  PreviewError_dot : Inport  Port=2
  HeadingError : Inport  Port=3
  HeadingError_dot : Inport  Port=4
  Curvature : Inport  Port=5
  Preview_Distance : Inport  Port=6
  Speed_m/s : Inport  Port=7
  Add : Sum  Inputs=++++
  Add1 : Sum
  Gain2 : Gain  Gain=0.0478
  Gain3 : Gain  Gain=-0.1
  Gain4 : Gain  Gain=0.1248
  Gain5 : Gain  Gain=0.0307
  Gain6 : Gain  Gain=0.015
  Gain7 : Gain  Gain=-1
  Gain8 : Gain  Gain=-0.2
  Integrator : Integrator
  LQR Feedforward : MATLAB Function  TreatAsAtomicUnit=on
  Scope : Scope  NumInputPorts=6
  Scope1 : Scope  NumInputPorts=2
  SteeringAngle_Front(rad) : Outport
  wires:
  PreviewError/1 -> Gain6/1, Gain2/1
  Gain4/1 -> Scope/3, Add/3
  Gain5/1 -> Scope/2, Add/2
  Gain3/1 -> Scope/4, Add/4
  Gain8/1 -> Scope/5, Add1/2, Scope1/2
  Gain2/1 -> Scope/1, Add/1
  Gain7/1 -> SteeringAngle_Front(rad)/1
  Add/1 -> Add1/1
  HeadingError_dot/1 -> Gain3/1
  Add1/1 -> Scope/6, Gain7/1
  Gain6/1 -> Integrator/1
  PreviewError_dot/1 -> Gain5/1
  HeadingError/1 -> Gain4/1
  Preview_Distance/1 -> LQR Feedforward/1(PreviewDistance)
  LQR Feedforward/1(Feedforward) -> Gain8/1
  Curvature/1 -> LQR Feedforward/2(Curvature)
  Integrator/1 -> Scope1/1
  Speed_m/s/1 -> LQR Feedforward/3(v)

== system Prescan_Carsim_1110_cs/BMW_X5_SUV_1/Tracking Control & vehicle dynamics/Lane Keeping Assistance/Path Tracking - LQR controller1 ==
  PreviewError : Inport
  PreviewError_dot : Inport  Port=2
  HeadingError : Inport  Port=3
  HeadingError_dot : Inport  Port=4
  Curvature : Inport  Port=5
  Preview_Distance : Inport  Port=6
  Speed_m/s : Inport  Port=7
  Add : Sum  Inputs=++++
  Add1 : Sum
  Gain2 : Gain  Gain=0.045
  Gain3 : Gain  Gain=-0.1
  Gain4 : Gain  Gain=0.1048
  Gain5 : Gain  Gain=0.0307
  Gain6 : Gain  Gain=0.015
  Gain7 : Gain  Gain=-1
  Gain8 : Gain  Gain=-0.08
  Integrator : Integrator
  LQR Feedforward : MATLAB Function  TreatAsAtomicUnit=on
  Scope : Scope  NumInputPorts=6
  Scope1 : Scope  NumInputPorts=2
  SteeringAngle_Front(rad) : Outport
  wires:
  PreviewError/1 -> Gain6/1, Gain2/1
  Gain4/1 -> Scope/3, Add/3
  Gain5/1 -> Scope/2, Add/2
  Gain3/1 -> Scope/4, Add/4
  Gain8/1 -> Scope/5, Add1/2, Scope1/2
  Gain2/1 -> Scope/1, Add/1
  Gain7/1 -> SteeringAngle_Front(rad)/1
  Add/1 -> Add1/1
  HeadingError_dot/1 -> Gain3/1
  Add1/1 -> Scope/6, Gain7/1
  Gain6/1 -> Integrator/1
  PreviewError_dot/1 -> Gain5/1
  HeadingError/1 -> Gain4/1
  Preview_Distance/1 -> LQR Feedforward/1(PreviewDistance)
  LQR Feedforward/1(Feedforward) -> Gain8/1
  Curvature/1 -> LQR Feedforward/2(Curvature)
  Integrator/1 -> Scope1/1
  Speed_m/s/1 -> LQR Feedforward/3(v)

== system Prescan_Carsim_1110_cs/BMW_X5_SUV_1/Tracking Control & vehicle dynamics/Lane Keeping Assistance/SMC characters ==
  note: 双移线和直线
  Abs : Abs
  Constant1 : Constant  Value=3.2
  Constant15 : Constant  Value=0.5
  Constant17 : Constant  Value=0.4
  Constant18 : Constant  Value=1.5
  Demux : Demux
  Display : Display
  Mux : Mux
  Mux1 : Mux
  Switch : Switch  Criteria=u2 > Threshold  Threshold=0.4
  st_angle_max10 : Constant  Value=3.5
  st_angle_max7 : Constant  Value=0.03
  st_angle_max8 : Constant  Value=2.3
  st_angle_max9 : Constant  Value=0.12
  tag scope: SMC_c1=global, SMC_c2=global, delta=global, kapa=global
  wires:
  Demux/1 -> [SMC_c1], Display/1
  st_angle_max7/1 -> Mux/3
  Constant18/1 -> Mux/1
  Demux/3 -> [delta]
  Mux/1 -> Switch/1
  [Lateral_Offset] -> Abs/1
  Demux/4 -> [kapa]
  Switch/1 -> Demux/1
  Constant1/1 -> Mux1/1
  Constant15/1 -> Mux/2
  Demux/2 -> [SMC_c2]
  st_angle_max9/1 -> Mux1/3
  Abs/1 -> Switch/2
  st_angle_max8/1 -> Mux/4
  st_angle_max10/1 -> Mux1/4
  Constant17/1 -> Mux1/2
  Mux1/1 -> Switch/3

== system Prescan_Carsim_1110_cs/BMW_X5_SUV_1/Tracking Control & vehicle dynamics/Lane Keeping Assistance/derivative_filter ==
  In1 : Inport
  Gain1 : Gain  Gain=0.8
  Gain2 : Gain  Gain=50
  Integrator2 : Integrator
  Sum1 : Sum  Inputs=|+-
  Out1 : Outport
  wires:
  Sum1/1 -> Gain2/1
  Integrator2/1 -> Sum1/2
  Gain1/1 -> Out1/1
  Gain2/1 -> Gain1/1, Integrator2/1
  In1/1 -> Sum1/1

== system Prescan_Carsim_1110_cs/BMW_X5_SUV_1/Tracking Control & vehicle dynamics/Lane Keeping Assistance/derivative_filter  ==
  In1 : Inport
  Gain1 : Gain  Gain=0.42
  Gain2 : Gain  Gain=40
  Integrator2 : Integrator
  Saturation : Saturate  UpperLimit=4  LowerLimit=-4
  Sum1 : Sum  Inputs=|+-
  Out1 : Outport
  wires:
  Saturation/1 -> Out1/1
  In1/1 -> Sum1/1
  Gain2/1 -> Integrator2/1, Gain1/1
  Integrator2/1 -> Sum1/2
  Sum1/1 -> Gain2/1
  Gain1/1 -> Saturation/1

== system Prescan_Carsim_1110_cs/BMW_X5_SUV_1/trajectory planning/A substitution for the above trajectory planning subsystem/Trajectory Planning For Curve under beginning-global ==
  note: The trajectory is a DataArray with 3 columns, the first two is the (X,Y) coordinates of the planed path ( under the vehicle coordinates system) , the third column is the planned velocity of that path point.
  RoadLane_Plan : Inport
  Parameter_TrajectoryPlan : Inport  Port=2
  VehicleWidth : Inport  Port=3
  LaneWidth : Inport  Port=4
  VehicleState_Global : Inport  Port=5
  Enable : EnablePort  PropagateVarSize=During execution
  Trigger : TriggerPort  VariantControl=Variant  PortDimensions=1
  LaneData_Gain2 : Gain
  Trajectory Planning For Curve : MATLAB Function  TreatAsAtomicUnit=on
  Path Plan : Outport
  Speed_Planned_kmh : Outport  Port=2
  PlanPathDataLength : Outport  Port=3
  VehicleState_CurvePlanningBeginning : Outport  Port=4  InitialOutput=[0 0 0]
  wires:
  Trajectory Planning For Curve/3(PlanPathDataLength_Curve) -> PlanPathDataLength/1
  LaneWidth/1 -> Trajectory Planning For Curve/4(LaneWidth)
  VehicleWidth/1 -> Trajectory Planning For Curve/3(VehicleWidth)
  VehicleState_Global/1 -> VehicleState_CurvePlanningBeginning/1
  RoadLane_Plan/1 -> LaneData_Gain2/1
  Trajectory Planning For Curve/1(Path_Plan) -> Path Plan/1
  Trajectory Planning For Curve/2(Speed_Planned_kmh) -> Speed_Planned_kmh/1
  Parameter_TrajectoryPlan/1 -> Trajectory Planning For Curve/2(Parameter_TrajectoryPlan)
  LaneData_Gain2/1 -> Trajectory Planning For Curve/1(RoadLane_Plan)

== system Prescan_Carsim_1110_cs/BMW_X5_SUV_1/trajectory planning/Specific Curve Trajectory Planning/Trajectory Planning For Curve under beginning-global ==
  note: The trajectory is a DataArray with 3 columns, the first two is the (X,Y) coordinates of the planed path ( under the vehicle coordinates system) , the third column is the planned velocity of that path point.
  RoadLane_Plan : Inport
  Parameter_TrajectoryPlan : Inport  Port=2
  VehicleWidth : Inport  Port=3
  LaneWidth : Inport  Port=4
  VehicleState_Global : Inport  Port=5
  Trigger : TriggerPort  VariantControl=Variant  InitialTriggerSignalState=negative  PortDimensions=1
  LaneData_Gain : Gain
  Trajectory Planning For Curve : MATLAB Function  TreatAsAtomicUnit=on
  Path Plan : Outport
  Speed_Planned_kmh : Outport  Port=2
  PlanPathDataLength : Outport  Port=3
  wires:
  Trajectory Planning For Curve/3(PlanPathDataLength_Curve) -> PlanPathDataLength/1
  LaneWidth/1 -> Trajectory Planning For Curve/4(LaneWidth)
  VehicleWidth/1 -> Trajectory Planning For Curve/3(VehicleWidth)
  VehicleState_Global/1 -> Trajectory Planning For Curve/5(VehicleState_Beginning)
  Trajectory Planning For Curve/2(Speed_Planned_kmh) -> Speed_Planned_kmh/1
  Parameter_TrajectoryPlan/1 -> Trajectory Planning For Curve/2(Parameter_TrajectoryPlan)
  RoadLane_Plan/1 -> LaneData_Gain/1
  Trajectory Planning For Curve/1(PathPlan_Global) -> Path Plan/1
  LaneData_Gain/1 -> Trajectory Planning For Curve/1(RoadLane_Plan)

== system Prescan_Carsim_1110_cs/BMW_X5_SUV_1/trajectory planning/Subsystem/Determination of Curve Road No ==
  Determine Curve No According the vehicle position : MATLAB Function  TreatAsAtomicUnit=on
      settings: AttributesFormatString=Curve 1:curve_length+60(30 meters befor and after curve)
  Curve No : Outport
  wires:
  [VehicleState_Global] -> Determine Curve No According the vehicle position/1(VehicleState_Global)
  Determine Curve No According the vehicle position/1(Curve_No) -> Curve No/1

== system Prescan_Carsim_1110_cs/BMW_X5_SUV_1/DEM updating and Preference Estimation/UpdateDEM/online DPM building preference estimation accordign to feedback/ Driver Perception Model preference to trajectory indicator ==
  "preference estimation " : Inport
  "Next Trajectory Sample Indicators " : Subsystem
  trajectory indicators : Outport
  wires:
  "preference estimation "/1 -> "Next Trajectory Sample Indicators "/1(In1)
  "Next Trajectory Sample Indicators "/1(Out1) -> trajectory indicators/1

== system Prescan_Carsim_1110_cs/BMW_X5_SUV_1/DEM updating and Preference Estimation/UpdateDEM/online DPM building preference estimation accordign to feedback/ Driver Perception Model preference to trajectory indicator/Next Trajectory Sample Indicators  ==
  In1 : Inport
  Out1 : Outport
  wires:
  In1/1 -> Out1/1
